simulink model "three_phase_inverter_pwm"  (Simulink 6.1)
settings: Solver=ode23tb  StartTime=0.0  StopTime=0.03  MaxStep=1e-5  RelTol=1e-3  AbsTol=.01
libraries: powerlib x14, simulink x1
settings Model: LastModifiedBy=ThinkPad
settings DebuggingCC: SolverPrmCheckMsg=warning

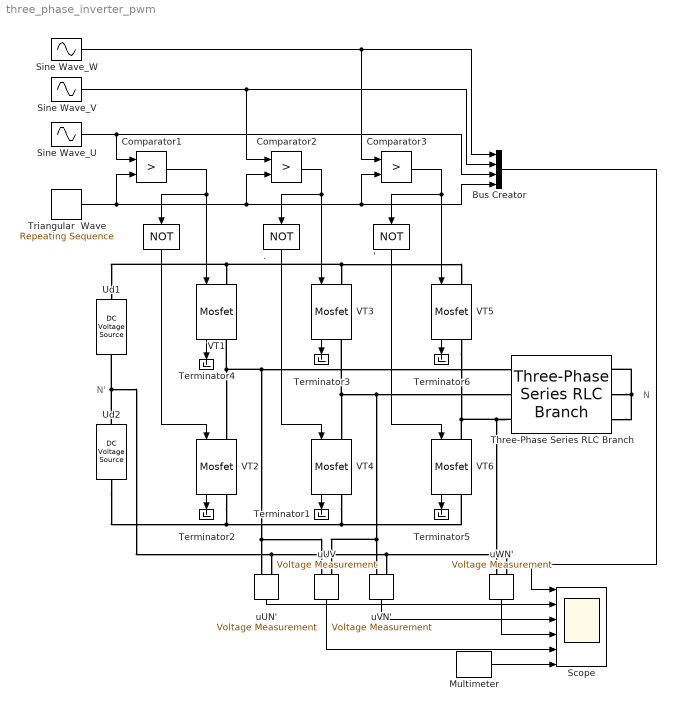
== system three_phase_inverter_pwm ==
  note: N'
  note: N
  " " : Logic  Orientation=down  Operator=NOT  AllPortsSameDT=off  OutDataTypeMode=Boolean
  " '" : Logic  Orientation=down  Operator=NOT  AllPortsSameDT=off  OutDataTypeMode=Boolean
  " ." : Logic  Orientation=down  Operator=NOT  AllPortsSameDT=off  OutDataTypeMode=Boolean
  Bus Creator : BusCreator  DialogController=Simulink.DDGSource_Bus
  Comparator1 : RelationalOperator  Operator=>  LogicOutDataTypeMode=Boolean  LogicDataType=sint(32)
  Comparator2 : RelationalOperator  Operator=>  LogicOutDataTypeMode=Boolean  LogicDataType=sint(32)
  Comparator3 : RelationalOperator  Operator=>  LogicOutDataTypeMode=Boolean  LogicDataType=sint(32)
  Multimeter : powerlib/Measurements/Multimeter  PhasorSimulation=off  OutputType=Complex  sel=1  L=6  Gain=1  yselected={'Ub1: Three-Phase Series RLC Branch'};  PSBOutputType=1  PSBequivalent=0  AxesSetting=[0,0.1,-100,100]  Display=0  SavedBlockNames=-11
  Scope : Scope  NumInputPorts=6
      settings: TimeRange=0.03  YMin=-1.5~-200~-200~-200~-300~-200  YMax=1.5~200~200~200~300~200  SampleTime=2e-4
  Sine Wave_U : Sin  Amplitude=0.7  Frequency=314  SampleTime=0
  Sine Wave_V : Sin  Amplitude=0.7  Frequency=314  Phase=-2*pi/3  SampleTime=0
  Sine Wave_W : Sin  Amplitude=0.7  Frequency=314  Phase=2*pi/3  SampleTime=0
  Terminator{1..6} (6 alike) : Terminator
      settings: Orientation=down
  Three-Phase Series RLC Branch : powerlib/Elements/Three-Phase Series RLC Branch  PhysicalDomain=powersysdomain  SubClassName=unknown  LeftPortType=p1  RightPortType=p1  LConnTagsString=A|B|C  RConnTagsString=A|B|C  Resistance=1  Inductance=0.005  Capacitance=inf  Measurements=Branch voltages and currents
  Triangular  Wave : simulink/Sources/Repeating Sequence  rep_seq_t=[0 2.5e-4 5e-4 7.5e-4 1e-3]  rep_seq_y=[0 1 0 -1 0]
  Ud1 : powerlib/Electrical Sources/DC Voltage Source  Orientation=up  Amplitude=100  Measurements=None
  Ud2 : powerlib/Electrical Sources/DC Voltage Source  Orientation=up  Amplitude=100  Measurements=None
  VT{1..6} (6 alike) : powerlib/Power Electronics/Mosfet  Orientation=down  Ron=0.01  Lon=1e-7  Rd=.01  IC=0  Rs=5  Cs=1e-6  Measurements=on
  uUN' : powerlib/Measurements/Voltage Measurement  Orientation=down  PhasorSimulation=off  OutputType=Complex  PSBequivalent=0
  uUV : powerlib/Measurements/Voltage Measurement  Orientation=down  PhasorSimulation=off  OutputType=Complex  PSBequivalent=0
  uVN' : powerlib/Measurements/Voltage Measurement  Orientation=down  PhasorSimulation=off  OutputType=Complex  PSBequivalent=0
  uWN' : powerlib/Measurements/Voltage Measurement  Orientation=down  PhasorSimulation=off  OutputType=Complex  PSBequivalent=0
  wires:
  Comparator1/1 -> " "/1, VT1/1
  VT4/1 -> Terminator1/1
  VT2/1 -> Terminator2/1
  VT3/1 -> Terminator3/1
  Sine Wave_U/1 -> Bus Creator/3, Comparator1/1
  Triangular  Wave/1 -> Comparator1/2, Comparator2/2, Comparator3/2, Bus Creator/4
  " "/1 -> VT2/1
  Multimeter/1 -> Scope/6
  VT1/1 -> Terminator4/1
  VT5/1 -> Terminator6/1
  VT6/1 -> Terminator5/1
  Comparator2/1 -> VT3/1, " ."/1
  Comparator3/1 -> VT5/1, " '"/1
  " ."/1 -> VT4/1
  " '"/1 -> VT6/1
  Sine Wave_V/1 -> Comparator2/1, Bus Creator/2
  Sine Wave_W/1 -> Comparator3/1, Bus Creator/1
  uUV/1 -> Scope/5
  uWN'/1 -> Scope/4
  uVN'/1 -> Scope/3
  uUN'/1 -> Scope/2
  Bus Creator/1 -> Scope/1
  connections:
  uUN'/LConn1 -- uUV/LConn1 -- Three-Phase Series RLC Branch/LConn1 -- VT1/RConn1 -- VT2/LConn1
  Ud2/LConn1 -- VT2/RConn1 -- VT6/RConn1 -- VT4/RConn1
  VT3/LConn1 -- VT5/LConn1 -- Ud1/RConn1 -- VT1/LConn1
  Three-Phase Series RLC Branch/LConn3 -- VT6/LConn1 -- VT5/RConn1 -- uWN'/LConn1
  Three-Phase Series RLC Branch/RConn2 -- Three-Phase Series RLC Branch/RConn3 -- Three-Phase Series RLC Branch/RConn1
  Ud2/RConn1 -- Ud1/LConn1 -- uUN'/LConn2 -- uWN'/LConn2 -- uVN'/LConn2
  VT3/RConn1 -- VT4/LConn1 -- Three-Phase Series RLC Branch/LConn2 -- uVN'/LConn1 -- uUV/LConn2
